simulink model "test_stateflow"  (R2020b)
settings: Solver=FixedStepAuto  StartTime=0.0  StopTime=N-time_step  FixedStep=time_step  RelTol=1e-3
values from neighbouring files (symbols this model uses):
  DEBOUNCE_TIME = 10*time_step    (= 10)    [StateTesting.m]
  S_inplane = ones(N,1)*[0 1 0]    [StateTesting.m]
  SLEW_LOWER = 0.05    [StateTesting.m]
  SLEW_UPPER = sind(30)    [StateTesting.m]
  time_step = 1    [AttitudeControlTesting.m]    (also in StateTesting.m)
  TUMBLE_LIMIT = 10    [StateTesting.m]
  v_ECI = [sin(angs) , cos(angs), zeros(N,1)]    [StateTesting.m]
  w = zeros(N,3)    [StateTesting.m]
settings Model: Creator=newpo  LastModifiedBy=newpo

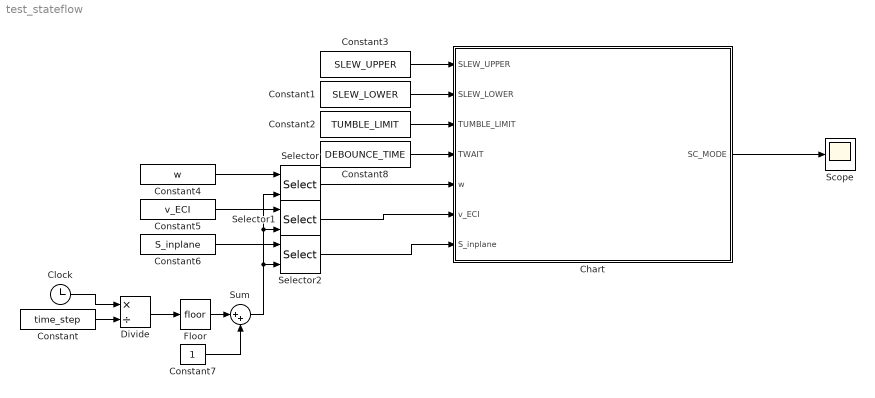
== system test_stateflow ==
  Chart : Stateflow chart  TreatAsAtomicUnit=on
  Clock : Clock
  Constant : Constant  Value=time_step
  Constant1 : Constant  Value=SLEW_LOWER
  Constant2 : Constant  Value=TUMBLE_LIMIT
  Constant3 : Constant  Value=SLEW_UPPER
  Constant4 : Constant  Value=w
  Constant5 : Constant  Value=v_ECI
  Constant6 : Constant  Value=S_inplane
  Constant7 : Constant
  Constant8 : Constant  Value=DEBOUNCE_TIME
  Divide : Product  Inputs=*/
  Floor : Rounding
  Scope : Scope
  Selector : Selector  NumberOfDimensions=2  InputPortWidth=3  IndexOptions=Index vector (port),Index vector (dialog)  Indices=[1 3],[1 2 3]  OutputSizes=1,1
  Selector1 : Selector  NumberOfDimensions=2  InputPortWidth=3  IndexOptions=Index vector (port),Index vector (dialog)  Indices=[1 3],[1 2 3]  OutputSizes=1,1
  Selector2 : Selector  NumberOfDimensions=2  InputPortWidth=3  IndexOptions=Index vector (port),Index vector (dialog)  Indices=[1 3],[1 2 3]  OutputSizes=1,1
  Sum : Sum  Inputs=|++
  wires:
  Selector1/1 -> Chart/6(v_ECI)
  Selector/1 -> Chart/5(w)
  Selector2/1 -> Chart/7(S_inplane)
  Clock/1 -> Divide/1
  Divide/1 -> Floor/1
  Sum/1 -> Selector/2, Selector1/2, Selector2/2
  Constant/1 -> Divide/2
  Constant4/1 -> Selector/1
  Constant5/1 -> Selector1/1
  Constant6/1 -> Selector2/1
  Constant1/1 -> Chart/2(SLEW_LOWER)
  Constant2/1 -> Chart/3(TUMBLE_LIMIT)
  Constant3/1 -> Chart/1(SLEW_UPPER)
  Floor/1 -> Sum/1
  Constant7/1 -> Sum/2
  Chart/1(SC_MODE) -> Scope/1
  Constant8/1 -> Chart/4(TWAIT)

== stateflow chart test_stateflow/Chart ==
  state SC_state [parallel]
    settings: executionOrder=1
    state stabilize
      entry:SC_MODE=STABILIZE;
    state slew
      entry: SC_MODE=SLEW;
    state detumble
      entry: SC_MODE = DETUMBLE;
    stabilize -> SC_state.slew [order 1] : Slew
    SC_state.slew -> stabilize [order 1] : Stabilize
    detumble -> stabilize : Stabilize
    stabilize -> detumble [order 2] : Detumble
    SC_state.slew -> detumble [order 2] : Detumble
    (default) -> detumble
  state SC_selectstate [parallel]
    settings: executionOrder=2
    state steady_state
    state stop_detumble
    state slew
    state do_detumble
    state start_detumble
    steady_state -> SC_selectstate.slew [order 2] : [abs(dot(v_ECI/norm(v_ECI),S_inplane))<SLEW_LOWER]
        | {send(Slew,SC_state)}
    stop_detumble -> steady_state [order 2] : after(TWAIT,sec)
        | [norm(w)<TUMBLE_LIMIT]
        | {send(Stabilize,SC_state)}
    SC_selectstate.slew -> steady_state [order 1] : [abs(dot(v_ECI/norm(v_ECI),S_inplane))>SLEW_UPPER]
        | {send(Stabilize,SC_state)}
    start_detumble -> steady_state [order 2] : [norm(w) < TUMBLE_LIMIT]
    steady_state -> start_detumble [order 1] : [norm(w) > TUMBLE_LIMIT]
    stop_detumble -> do_detumble [order 1] : [norm(w) > TUMBLE_LIMIT]
    do_detumble -> stop_detumble : [norm(w) < TUMBLE_LIMIT]
    SC_selectstate.slew -> start_detumble [order 2] : [norm(w) > TUMBLE_LIMIT]
    (default) -> do_detumble
    start_detumble -> do_detumble [order 1] : after(TWAIT,sec)
        | [norm(w)>TUMBLE_LIMIT]
        | {send(Detumble,SC_state)}
  data: SLEW_UPPER input; SLEW_LOWER input; TUMBLE_LIMIT input; TWAIT input =1; w input; v_ECI input; S_inplane input; SC_MODE output Enum: SCModeEnum
  events: Stabilize local FUNCTION_CALL_EVENT; Slew local FUNCTION_CALL_EVENT; Detumble local FUNCTION_CALL_EVENT
